simulink model "Current_Fed_DC_DC_Converter_Code_Equivalent_v4"  (R2020a)
settings: Solver=ode3  StartTime=0.0  StopTime=0.4  MaxStep=1e-5  MinStep=1e-7  RelTol=1e-6
InitFcn:
  | %Supply
  | V_supply = 415;
  | f_supply = 50;
  | 
  | %DC_Bus
  | C_filt = 220e-6
  | L_dc = 100e-6;
  | C_out = 560e-3;
  | 
  | %Transformer
  | P_TX = 10e3;
  | V_pri = 36;
  | V_sec = 1;
  | L_leak = 0;
  | R_leak = 0;
  | L_mag = inf;
  | R_mag = inf;
  | 
  | %Control
  | f_sw = 15e3;
  | tss_conv = 0.1;
  | V_ref = 1480;
  | Kp_V = 1;
  | Ki_V = 0.001;
  | I_ref = 2920;
  | Kp_I = 0.025;
  | Ki_I = 0.000001;
  | PS_max = 180;
  | Carr_offset = 1;
  | Carr_scale = 0.5;
  | Duty_scale = 0.01;
  | Duty_fix = 50;
  | Duty_max = 75;
  | Duty_min = 0;
  | f_chop = 1e3;
  | Duty_chop = 40;
  | 
  | %Harmonic_Correction
  | P_inj = 50;
  | f_inj = 50;
  | L_inj = 10e-6;
  | R_inj = 1;
  | Vpri_inj = 1;
  | Vsec_inj = 70;
  | Rleak_inj = 1e-3;
  | Lleak_inj = 12e-6;
  | R_inj = 0.1;
  | Rmag_inj = 1e-3;
  | Lmag_inj = 1e-3;
  | 
  | %Sensor
  | ADC_Res = 4096;
  | I_sense = 1/700;
  | V_sense = 1/50;
  | 
  | %Faults
  | OV_limit = 18.25;
  | UV_limit = 17.5;
  | OC_limit = 515;
  | UC_limit = 22;
  | ... (+3 lines)
libraries: powerlib x109, powerlib_meascontrol x30, simulink x5, slctrlblks x2
(part 2 of 3)

== system Current_Fed_DC_DC_Converter_Code_Equivalent_v4/Module 2/DC DC Converter/DC Bus ==
  DC Bus Parameter : Scope  Commented=on  NumInputPorts=2
  Idc filt : powerlib/Measurements/Current Measurement  PhasorSimulation=off  OutputType=Complex  PSBequivalent=0
  L bus : powerlib/Elements/Series RLC Branch  LConnTagsString=__new0  RConnTagsString=__new0  BranchType=L  Resistance=1  Inductance=L_dc  SetiL0=off  InitialCurrent=0  Capacitance=1e-6  Setx0=off  InitialVoltage=0  Measurements=None
  Vdc : powerlib/Measurements/Voltage Measurement  PhasorSimulation=off  OutputType=Complex  PSBequivalent=0
  +ve IN : PMIOPort  Side=Left
  -ve IN : PMIOPort  Port=2  Side=Left
  +ve OUT : PMIOPort  Port=3  Side=Right
  -ve OUT : PMIOPort  Port=4  Side=Right
  wires:
  Vdc/1 -> DC Bus Parameter/2  "Vdc"
  Idc filt/1 -> DC Bus Parameter/1  "Ifilt"
  connections:
  Idc filt/RConn1 -- +ve OUT/RConn1
  Idc filt/LConn1 -- Vdc/LConn1 -- L bus/RConn1
  Vdc/LConn2 -- -ve IN/RConn1 -- -ve OUT/RConn1
  +ve IN/RConn1 -- L bus/LConn1

== system Current_Fed_DC_DC_Converter_Code_Equivalent_v4/Module 2/DC DC Converter/Filter ==
  C out : powerlib/Elements/Series RLC Branch  LConnTagsString=__new0  RConnTagsString=__new0  BranchType=C  Resistance=10  Inductance=1e-3  SetiL0=off  InitialCurrent=0  Capacitance=C_out  Setx0=off  InitialVoltage=0  Measurements=None
  I C Filter : powerlib/Measurements/Current Measurement  PhasorSimulation=off  OutputType=Complex  PSBequivalent=0
  I out : powerlib/Measurements/Current Measurement  PhasorSimulation=off  OutputType=Complex  PSBequivalent=0
  Output Filter Parameters : Scope  Commented=on  NumInputPorts=2
  +ve IN : PMIOPort  Side=Left
  -ve IN : PMIOPort  Port=2  Side=Left
  +ve OUT : PMIOPort  Port=3  Side=Right
  -ve OUT : PMIOPort  Port=4  Side=Right
  wires:
  I C Filter/1 -> Output Filter Parameters/2
  I out/1 -> Output Filter Parameters/1
  connections:
  +ve OUT/RConn1 -- I out/RConn1
  I C Filter/RConn1 -- C out/LConn1
  I C Filter/LConn1 -- +ve IN/RConn1 -- I out/LConn1
  C out/RConn1 -- -ve OUT/RConn1 -- -ve IN/RConn1

== system Current_Fed_DC_DC_Converter_Code_Equivalent_v4/Module 2/DC DC Converter/HF Transformer ==
  Centre-Tap Transformer 40:1 : powerlib/Elements/Linear Transformer  UNITS=SI  NominalPower=[P_TX f_sw]  winding1=[V_pri R_leak L_leak]  winding2=[V_sec R_leak L_leak]  ThreeWindings=on  winding3=[V_sec R_leak L_leak]  RmLm=[R_mag L_mag]  Measurements=None  DataType=on
  High Frequency Transformer Parameters : Scope  Commented=on  NumInputPorts=5
  Ipri : powerlib/Measurements/Current Measurement  PhasorSimulation=off  OutputType=Complex  PSBequivalent=0
  Isec : powerlib/Measurements/Current Measurement  PhasorSimulation=off  OutputType=Complex  PSBequivalent=0
  Vpri : powerlib/Measurements/Voltage Measurement  PhasorSimulation=off  OutputType=Complex  PSBequivalent=0
  Vsec1 : powerlib/Measurements/Voltage Measurement  PhasorSimulation=off  OutputType=Complex  PSBequivalent=0
  Vsec2 : powerlib/Measurements/Voltage Measurement  PhasorSimulation=off  OutputType=Complex  PSBequivalent=0
  L pri : PMIOPort  Side=Left
  N pri : PMIOPort  Port=2  Side=Left
  L sec : PMIOPort  Port=3  Side=Right
  CT : PMIOPort  Port=4  Side=Right
  N sec : PMIOPort  Port=5  Side=Right
  wires:
  Vpri/1 -> High Frequency Transformer Parameters/5  "V primary"
  Ipri/1 -> High Frequency Transformer Parameters/4  "I primary"
  Vsec2/1 -> High Frequency Transformer Parameters/3  "V secondary 2"
  Vsec1/1 -> High Frequency Transformer Parameters/2  "V secondary 1"
  Isec/1 -> High Frequency Transformer Parameters/1  "I secondary"
  connections:
  Centre-Tap Transformer 40:1/RConn1 -- Vsec1/LConn1 -- Isec/LConn1
  Isec/RConn1 -- L sec/RConn1
  Centre-Tap Transformer 40:1/LConn1 -- Ipri/RConn1
  Centre-Tap Transformer 40:1/RConn4 -- Vsec2/LConn2 -- N sec/RConn1
  Centre-Tap Transformer 40:1/RConn3 -- Centre-Tap Transformer 40:1/RConn2 -- Vsec2/LConn1 -- Vsec1/LConn2 -- CT/RConn1
  Vpri/LConn1 -- L pri/RConn1 -- Ipri/LConn1
  N pri/RConn1 -- Vpri/LConn2 -- Centre-Tap Transformer 40:1/LConn2

== system Current_Fed_DC_DC_Converter_Code_Equivalent_v4/Module 2/DC DC Converter/Inverter ==
  Iref : Inport
  Ifeed : Inport  Port=2
  Vfeed : Inport  Port=3
  Converter : Subsystem
      settings: PortSchema="{\"entries\":[{\"content\":{\"sides\":[{\"content\":{\"connectorIds\":[\"LConn1\",\"LConn2\"]},\"type\":\"ConnectorPlacement.EquallySpacedRectSide\",\"uuid\":\"0645cdc9-e655-49ab-a1d8-1293a5a1d66e\"},{\"content\":{\"connectorIds\":[\"RConn1\",\"RConn2\"],\"side\":\"RIGHT\"},\"type\":\"ConnectorPlacement.EquallySpacedRectSide\",\"uuid\":\"2ef7d2b0-2c84-4192-a188-141ae61cdfda\"},{\"content\":{\"connectorIds\":[\"In1\"],\"side\":\"TOP\"},\"type\":\"ConnectorPlacement.EquallySpacedRectSide\",\"uuid\":\"c5fd5dee-0ba9-4cec-8a2b-47382b263168\"}]},\"type\":\"ConnectorPlacement.EquallySpacedConnector\",\"uuid\":\"4d765392-2146-4c23-badc-b27487fa349e\"}],\"packageUris\":[\"http://schema.mathworks.com/mf0/Connector/19700101\"],\"version\":\"1.0\"}"
  Pulse Generator : Subsystem
  +ve : PMIOPort  Side=Left
  -ve : PMIOPort  Port=2  Side=Left
  Line : PMIOPort  Port=3  Side=Right
  Neutral : PMIOPort  Port=4  Side=Right
  Iref Main : Outport
  wires:
  Iref/1 -> Pulse Generator/1(Iref)
  Pulse Generator/2(Iref Main) -> Iref Main/1
  Ifeed/1 -> Pulse Generator/2(I feed)
  Pulse Generator/1(Pulses) -> Converter/1(Pulses)
  Vfeed/1 -> Pulse Generator/3(V Feed)
  connections:
  Converter/RConn2 -- Neutral/RConn1
  Converter/RConn1 -- Line/RConn1
  Converter/LConn1 -- +ve/RConn1
  Converter/LConn2 -- -ve/RConn1

== system Current_Fed_DC_DC_Converter_Code_Equivalent_v4/Module 2/DC DC Converter/Sensor ==
  Iin : Inport
  Vin : Inport  Port=2
  Current 12bit ADC : Gain  Gain=ADC_Res
  Current Transducer : Gain  Gain=I_sense
  Voltage 12bit ADC : Gain  Gain=ADC_Res
  Voltage Transducer : Gain  Gain=V_sense
  Iout : Outport
  Vout : Outport  Port=2
  wires:
  Vin/1 -> Voltage Transducer/1
  Voltage 12bit ADC/1 -> Vout/1
  Current 12bit ADC/1 -> Iout/1
  Voltage Transducer/1 -> Voltage 12bit ADC/1
  Current Transducer/1 -> Current 12bit ADC/1
  Iin/1 -> Current Transducer/1

== system Current_Fed_DC_DC_Converter_Code_Equivalent_v4/Module 3/3 Phase Rectifier/3 Phase Rectifier ==
  D{1..6} (6 alike) : powerlib/Power Electronics/Diode  Ron=0.001  Lon=0  Vf=0.8  IC=0  UseSnubber=0  Rs=500  Cs=250e-9  Measurements=on
  D1 V&I : Scope  Commented=on
  D2 V&I : Scope  Commented=on
  D3 V&I : Scope  Commented=on
  D4 V&I : Scope  Commented=on
  D5 V&I : Scope  Commented=on
  D6 V&I : Scope  Commented=on
  R Phase : PMIOPort  Side=Left
  Y Phase : PMIOPort  Port=2  Side=Left
  B Phase : PMIOPort  Port=3  Side=Left
  +ve : PMIOPort  Port=4  Side=Right
  -ve : PMIOPort  Port=5  Side=Right
  wires:
  D1/1 -> D1 V&I/1
  D4/1 -> D4 V&I/1
  D3/1 -> D3 V&I/1
  D5/1 -> D5 V&I/1
  D2/1 -> D2 V&I/1
  D6/1 -> D6 V&I/1
  connections:
  B Phase/RConn1 -- D2/RConn1 -- D5/LConn1
  Y Phase/RConn1 -- D4/RConn1 -- D3/LConn1
  -ve/RConn1 -- D2/LConn1 -- D4/LConn1 -- D6/LConn1
  D5/RConn1 -- +ve/RConn1 -- D3/RConn1 -- D1/RConn1
  R Phase/RConn1 -- D6/RConn1 -- D1/LConn1

== system Current_Fed_DC_DC_Converter_Code_Equivalent_v4/Module 3/3 Phase Rectifier/Filter ==
  Cdc 1 : powerlib/Elements/Series RLC Branch  LConnTagsString=__new0  RConnTagsString=__new0  BranchType=C  Resistance=1  Inductance=1e-3  SetiL0=off  InitialCurrent=0  Capacitance=2*C_filt  Setx0=off  InitialVoltage=0  Measurements=None
  Cdc 2 : powerlib/Elements/Series RLC Branch  LConnTagsString=__new0  RConnTagsString=__new0  BranchType=C  Resistance=1  Inductance=1e-3  SetiL0=off  InitialCurrent=0  Capacitance=2*C_filt  Setx0=off  InitialVoltage=0  Measurements=None
  DC Bus Filter Parameters : Scope  NumInputPorts=2
  Iout : powerlib/Measurements/Current Measurement  PhasorSimulation=off  OutputType=Complex  PSBequivalent=0
  Vout : powerlib/Measurements/Voltage Measurement  PhasorSimulation=off  OutputType=Complex  PSBequivalent=0
  +ve IN : PMIOPort  Side=Left
  -ve In : PMIOPort  Port=2  Side=Left
  +ve OUT : PMIOPort  Port=3  Side=Right
  Mid : PMIOPort  Port=4  Side=Right
  -ve OUT : PMIOPort  Port=5  Side=Right
  wires:
  Vout/1 -> DC Bus Filter Parameters/2  "Vout"
  Iout/1 -> DC Bus Filter Parameters/1  "Iout"
  connections:
  Mid/RConn1 -- Cdc 2/LConn1 -- Cdc 1/RConn1
  +ve OUT/RConn1 -- Iout/RConn1
  -ve OUT/RConn1 -- -ve In/RConn1 -- Cdc 2/RConn1 -- Vout/LConn2
  Iout/LConn1 -- +ve IN/RConn1 -- Cdc 1/LConn1 -- Vout/LConn1

== system Current_Fed_DC_DC_Converter_Code_Equivalent_v4/Module 3/DC DC Converter/Centre Tap Rectifier ==
  D1 : powerlib/Power Electronics/Diode  Ron=0.001  Lon=0  Vf=0.8  IC=0  UseSnubber=0  Rs=500  Cs=250e-9  Measurements=on
  D1 V&I : Scope  Commented=on
  D2 : powerlib/Power Electronics/Diode  Ron=0.001  Lon=0  Vf=0.8  IC=0  UseSnubber=0  Rs=500  Cs=250e-9  Measurements=on
  D2 V&I1 : Scope  Commented=on
  Line : PMIOPort  Side=Left
  Centre-tap : PMIOPort  Port=2  Side=Left
  Neutral : PMIOPort  Port=3  Side=Left
  +ve : PMIOPort  Port=4  Side=Right
  -ve : PMIOPort  Port=5  Side=Right
  wires:
  D1/1 -> D1 V&I/1
  D2/1 -> D2 V&I1/1
  connections:
  D1/RConn1 -- +ve/RConn1 -- D2/RConn1
  D1/LConn1 -- Line/RConn1
  D2/LConn1 -- Neutral/RConn1
  -ve/RConn1 -- Centre-tap/RConn1

== system Current_Fed_DC_DC_Converter_Code_Equivalent_v4/Module 3/DC DC Converter/Chopper ==
  Chop Pulse Generator : Subsystem
  Fault Detection : Subsystem
  Io avg : powerlib_meascontrol/Measurements/Mean  Freq=f_supply  Vinit=0  Ts=0
  Iout : powerlib/Measurements/Current Measurement  PhasorSimulation=off  OutputType=Complex  PSBequivalent=0
  Out Parameters : Scope  NumInputPorts=2
  Qchop : powerlib/Power Electronics/IGBT  Ron=0.001  Lon=0  Vf=1  Tf=1e-6  Tt=2e-6  IC=0  Rs=1e5  Cs=inf  Measurements=on
  Qchop V&I : Scope  Commented=on
  Rchop : powerlib/Elements/Series RLC Branch  LConnTagsString=__new0  RConnTagsString=__new0  BranchType=R  Resistance=0.1  Inductance=1e-3  SetiL0=off  InitialCurrent=0  Capacitance=1e-6  Setx0=off  InitialVoltage=0  Measurements=None
  Vo avg : powerlib_meascontrol/Measurements/Mean  Freq=f_supply  Vinit=0  Ts=0
  Vout : powerlib/Measurements/Voltage Measurement  PhasorSimulation=off  OutputType=Complex  PSBequivalent=0
  +ve IN : PMIOPort  Side=Left
  -ve IN : PMIOPort  Port=2  Side=Left
  +ve OUT : PMIOPort  Port=3  Side=Right
  -ve OUT : PMIOPort  Port=4  Side=Right
  Idc avg : Outport
  Vdc avg : Outport  Port=2
  Vdc : Outport  Port=3
  " Idc" : Outport  Port=4
  wires:
  Chop Pulse Generator/1(Chop Pulse) -> Qchop/1
  Vo avg/1 -> Vdc avg/1  "Vo avg"
  Qchop/1 -> Qchop V&I/1
  Iout/1 -> " Idc"/1, Fault Detection/2(I Output), Io avg/1, Out Parameters/1  "Iout"
  Io avg/1 -> Idc avg/1  "Io avg"
  Vout/1 -> Vdc/1, Vo avg/1, Out Parameters/2, Fault Detection/1(V Output)  "Vout"
  Fault Detection/1(OV Fault) -> Chop Pulse Generator/1(Over Voltage Fault)
  connections:
  +ve OUT/RConn1 -- Iout/RConn1 -- Vout/LConn1
  Rchop/LConn1 -- Qchop/RConn1
  Iout/LConn1 -- +ve IN/RConn1 -- Qchop/LConn1
  -ve OUT/RConn1 -- -ve IN/RConn1 -- Rchop/RConn1 -- Vout/LConn2

== system Current_Fed_DC_DC_Converter_Code_Equivalent_v4/Module 3/DC DC Converter/DC Bus ==
  DC Bus Parameter : Scope  Commented=on  NumInputPorts=2
  Idc filt : powerlib/Measurements/Current Measurement  PhasorSimulation=off  OutputType=Complex  PSBequivalent=0
  L bus : powerlib/Elements/Series RLC Branch  LConnTagsString=__new0  RConnTagsString=__new0  BranchType=L  Resistance=1  Inductance=L_dc  SetiL0=off  InitialCurrent=0  Capacitance=1e-6  Setx0=off  InitialVoltage=0  Measurements=None
  Vdc : powerlib/Measurements/Voltage Measurement  PhasorSimulation=off  OutputType=Complex  PSBequivalent=0
  +ve IN : PMIOPort  Side=Left
  -ve IN : PMIOPort  Port=2  Side=Left
  +ve OUT : PMIOPort  Port=3  Side=Right
  -ve OUT : PMIOPort  Port=4  Side=Right
  wires:
  Vdc/1 -> DC Bus Parameter/2  "Vdc"
  Idc filt/1 -> DC Bus Parameter/1  "Ifilt"
  connections:
  Idc filt/RConn1 -- +ve OUT/RConn1
  Idc filt/LConn1 -- Vdc/LConn1 -- L bus/RConn1
  Vdc/LConn2 -- -ve IN/RConn1 -- -ve OUT/RConn1
  +ve IN/RConn1 -- L bus/LConn1

== system Current_Fed_DC_DC_Converter_Code_Equivalent_v4/Module 3/DC DC Converter/Filter ==
  C out : powerlib/Elements/Series RLC Branch  LConnTagsString=__new0  RConnTagsString=__new0  BranchType=C  Resistance=10  Inductance=1e-3  SetiL0=off  InitialCurrent=0  Capacitance=C_out  Setx0=off  InitialVoltage=0  Measurements=None
  I C Filter : powerlib/Measurements/Current Measurement  PhasorSimulation=off  OutputType=Complex  PSBequivalent=0
  I out : powerlib/Measurements/Current Measurement  PhasorSimulation=off  OutputType=Complex  PSBequivalent=0
  Output Filter Parameters : Scope  Commented=on  NumInputPorts=2
  +ve IN : PMIOPort  Side=Left
  -ve IN : PMIOPort  Port=2  Side=Left
  +ve OUT : PMIOPort  Port=3  Side=Right
  -ve OUT : PMIOPort  Port=4  Side=Right
  wires:
  I C Filter/1 -> Output Filter Parameters/2
  I out/1 -> Output Filter Parameters/1
  connections:
  +ve OUT/RConn1 -- I out/RConn1
  I C Filter/RConn1 -- C out/LConn1
  I C Filter/LConn1 -- +ve IN/RConn1 -- I out/LConn1
  C out/RConn1 -- -ve OUT/RConn1 -- -ve IN/RConn1

== system Current_Fed_DC_DC_Converter_Code_Equivalent_v4/Module 3/DC DC Converter/HF Transformer ==
  Centre-Tap Transformer 40:1 : powerlib/Elements/Linear Transformer  UNITS=SI  NominalPower=[P_TX f_sw]  winding1=[V_pri R_leak L_leak]  winding2=[V_sec R_leak L_leak]  ThreeWindings=on  winding3=[V_sec R_leak L_leak]  RmLm=[R_mag L_mag]  Measurements=None  DataType=on
  High Frequency Transformer Parameters : Scope  Commented=on  NumInputPorts=5
  Ipri : powerlib/Measurements/Current Measurement  PhasorSimulation=off  OutputType=Complex  PSBequivalent=0
  Isec : powerlib/Measurements/Current Measurement  PhasorSimulation=off  OutputType=Complex  PSBequivalent=0
  Vpri : powerlib/Measurements/Voltage Measurement  PhasorSimulation=off  OutputType=Complex  PSBequivalent=0
  Vsec1 : powerlib/Measurements/Voltage Measurement  PhasorSimulation=off  OutputType=Complex  PSBequivalent=0
  Vsec2 : powerlib/Measurements/Voltage Measurement  PhasorSimulation=off  OutputType=Complex  PSBequivalent=0
  L pri : PMIOPort  Side=Left
  N pri : PMIOPort  Port=2  Side=Left
  L sec : PMIOPort  Port=3  Side=Right
  CT : PMIOPort  Port=4  Side=Right
  N sec : PMIOPort  Port=5  Side=Right
  wires:
  Vpri/1 -> High Frequency Transformer Parameters/5  "V primary"
  Ipri/1 -> High Frequency Transformer Parameters/4  "I primary"
  Vsec2/1 -> High Frequency Transformer Parameters/3  "V secondary 2"
  Vsec1/1 -> High Frequency Transformer Parameters/2  "V secondary 1"
  Isec/1 -> High Frequency Transformer Parameters/1  "I secondary"
  connections:
  Centre-Tap Transformer 40:1/RConn1 -- Vsec1/LConn1 -- Isec/LConn1
  Isec/RConn1 -- L sec/RConn1
  Centre-Tap Transformer 40:1/LConn1 -- Ipri/RConn1
  Centre-Tap Transformer 40:1/RConn4 -- Vsec2/LConn2 -- N sec/RConn1
  Centre-Tap Transformer 40:1/RConn3 -- Centre-Tap Transformer 40:1/RConn2 -- Vsec2/LConn1 -- Vsec1/LConn2 -- CT/RConn1
  Vpri/LConn1 -- L pri/RConn1 -- Ipri/LConn1
  N pri/RConn1 -- Vpri/LConn2 -- Centre-Tap Transformer 40:1/LConn2

== system Current_Fed_DC_DC_Converter_Code_Equivalent_v4/Module 3/DC DC Converter/Inverter ==
  Iref : Inport
  Ifeed : Inport  Port=2
  Vfeed : Inport  Port=3
  Converter : Subsystem
      settings: PortSchema="{\"entries\":[{\"content\":{\"sides\":[{\"content\":{\"connectorIds\":[\"LConn1\",\"LConn2\"]},\"type\":\"ConnectorPlacement.EquallySpacedRectSide\",\"uuid\":\"0645cdc9-e655-49ab-a1d8-1293a5a1d66e\"},{\"content\":{\"connectorIds\":[\"RConn1\",\"RConn2\"],\"side\":\"RIGHT\"},\"type\":\"ConnectorPlacement.EquallySpacedRectSide\",\"uuid\":\"2ef7d2b0-2c84-4192-a188-141ae61cdfda\"},{\"content\":{\"connectorIds\":[\"In1\"],\"side\":\"TOP\"},\"type\":\"ConnectorPlacement.EquallySpacedRectSide\",\"uuid\":\"c5fd5dee-0ba9-4cec-8a2b-47382b263168\"}]},\"type\":\"ConnectorPlacement.EquallySpacedConnector\",\"uuid\":\"4d765392-2146-4c23-badc-b27487fa349e\"}],\"packageUris\":[\"http://schema.mathworks.com/mf0/Connector/19700101\"],\"version\":\"1.0\"}"
  Pulse Generator : Subsystem
  +ve : PMIOPort  Side=Left
  -ve : PMIOPort  Port=2  Side=Left
  Line : PMIOPort  Port=3  Side=Right
  Neutral : PMIOPort  Port=4  Side=Right
  Iref Main : Outport
  wires:
  Iref/1 -> Pulse Generator/1(Iref)
  Pulse Generator/2(Iref Main) -> Iref Main/1
  Ifeed/1 -> Pulse Generator/2(I feed)
  Pulse Generator/1(Pulses) -> Converter/1(Pulses)
  Vfeed/1 -> Pulse Generator/3(V Feed)
  connections:
  Converter/RConn2 -- Neutral/RConn1
  Converter/RConn1 -- Line/RConn1
  Converter/LConn1 -- +ve/RConn1
  Converter/LConn2 -- -ve/RConn1

== system Current_Fed_DC_DC_Converter_Code_Equivalent_v4/Module 3/DC DC Converter/Sensor ==
  Iin : Inport
  Vin : Inport  Port=2
  Current 12bit ADC : Gain  Gain=ADC_Res
  Current Transducer : Gain  Gain=I_sense
  Voltage 12bit ADC : Gain  Gain=ADC_Res
  Voltage Transducer : Gain  Gain=V_sense
  Iout : Outport
  Vout : Outport  Port=2
  wires:
  Vin/1 -> Voltage Transducer/1
  Voltage 12bit ADC/1 -> Vout/1
  Current 12bit ADC/1 -> Iout/1
  Voltage Transducer/1 -> Voltage 12bit ADC/1
  Current Transducer/1 -> Current 12bit ADC/1
  Iin/1 -> Current Transducer/1

== system Current_Fed_DC_DC_Converter_Code_Equivalent_v4/Module 1/DC DC Converter/Chopper/Chop Pulse Generator ==
  Over Voltage Fault : Inport
  Carrier Bias : Constant  Value=Carr_offset
  Carrier Scaling : Gain  Gain=Carr_scale
  Chopping Carrier : powerlib_meascontrol/Pulse & Signal Generators/Sawtooth Generator  Freq=f_chop  Phase=0  Ts=0
  Chopping Duty Cycle : Constant  Value=Duty_chop
  Chopping Pulse Parameters : Scope  Commented=on  NumInputPorts=4
  Comparator : RelationalOperator  Operator=<=  OutDataTypeStr=boolean  RndMeth=Simplest
  Duty Cycle Scaling : Gain  Gain=Duty_scale
  Fault Condition Check : Logic  IconShape=distinctive  AllPortsSameDT=off  OutDataTypeStr=boolean
  Level Correction : Sum  Inputs=|++
  Chop Pulse : Outport
  wires:
  Chopping Duty Cycle/1 -> Duty Cycle Scaling/1
  Fault Condition Check/1 -> Chop Pulse/1, Chopping Pulse Parameters/4  "Chop Pulse"
  Level Correction/1 -> Carrier Scaling/1
  Duty Cycle Scaling/1 -> Comparator/2
  Carrier Scaling/1 -> Chopping Pulse Parameters/1, Comparator/1  "Chopper Carrier Wave"
  Over Voltage Fault/1 -> Chopping Pulse Parameters/3, Fault Condition Check/2  "Over-voltage Fault"
  Carrier Bias/1 -> Level Correction/2
  Comparator/1 -> Chopping Pulse Parameters/2, Fault Condition Check/1  "Generic Pulse"
  Chopping Carrier/1 -> Level Correction/1

== system Current_Fed_DC_DC_Converter_Code_Equivalent_v4/Module 1/DC DC Converter/Chopper/Fault Detection ==
  V Output : Inport
  I Output : Inport  Port=2
  Constant : Constant  Value=OV_limit
  Constant1 : Constant  Value=UV_limit
  Constant2 : Constant  Value=OC_limit
  Constant3 : Constant  Value=UC_limit
  Faults : Scope  Commented=on  NumInputPorts=4
  GreaterThan : RelationalOperator  OutDataTypeStr=boolean  RndMeth=Simplest
  GreaterThan1 : RelationalOperator  Operator=<=  OutDataTypeStr=boolean  RndMeth=Simplest
  GreaterThan2 : RelationalOperator  OutDataTypeStr=boolean  RndMeth=Simplest
  GreaterThan3 : RelationalOperator  Operator=<=  OutDataTypeStr=boolean  RndMeth=Simplest
  OV Fault : Outport
  wires:
  Constant2/1 -> GreaterThan2/2
  V Output/1 -> GreaterThan1/1, GreaterThan/1
  Constant/1 -> GreaterThan/2
  Constant3/1 -> GreaterThan3/2
  I Output/1 -> GreaterThan2/1, GreaterThan3/1
  GreaterThan3/1 -> Faults/4  "Under Current Fault"
  Constant1/1 -> GreaterThan1/2
  GreaterThan1/1 -> Faults/2  "Under Voltage Fault"
  GreaterThan2/1 -> Faults/3  "Over Current Fault"
  GreaterThan/1 -> OV Fault/1, Faults/1  "Over Voltage Fault"

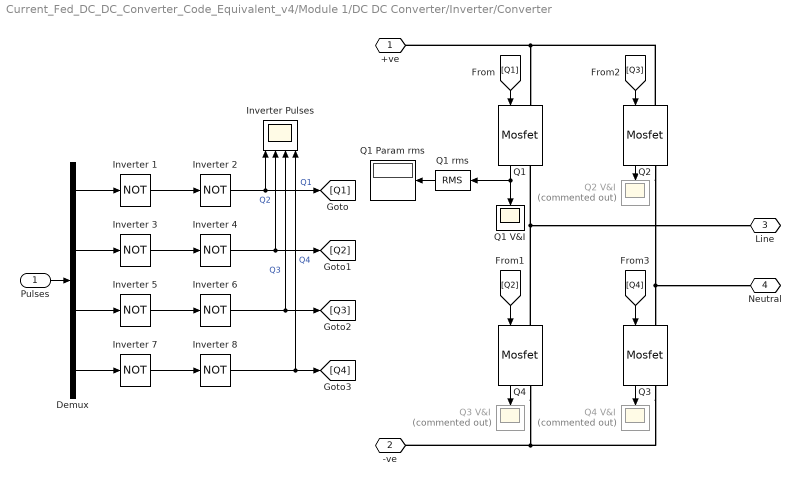
== system Current_Fed_DC_DC_Converter_Code_Equivalent_v4/Module 1/DC DC Converter/Inverter/Converter ==
  Pulses : Inport
  Demux : Demux
  Inverter Pulses : Scope  NumInputPorts=4
  Inverter {1..8} (8 alike) : Logic  Operator=NOT  IconShape=distinctive  AllPortsSameDT=off  OutDataTypeStr=boolean
  Q{1..4} (4 alike) : powerlib/Power Electronics/Mosfet  Ron=0.1  Lon=0  Rd=0.01  Vfd=0  IC=0  Rs=1e5  Cs=inf  Measurements=on
  Q1 V&I : Scope
  Q1 Param rms : Display
  Q1 rms : powerlib_meascontrol/Measurements/RMS  TrueRMS=on  Freq=f_supply  RMSInit=0  Ts=0
  Q2 V&I : Scope  Commented=on
  Q3 V&I : Scope  Commented=on
  Q4 V&I : Scope  Commented=on
  +ve : PMIOPort  Side=Left
  -ve : PMIOPort  Port=2  Side=Left
  Line : PMIOPort  Port=3  Side=Right
  Neutral : PMIOPort  Port=4  Side=Right
  wires:
  Pulses/1 -> Demux/1
  Demux/4 -> Inverter 7/1
  [Q3] -> Q2/1
  [Q1] -> Q1/1
  [Q4] -> Q3/1
  Q4/1 -> Q3 V&I/1
  Q3/1 -> Q4 V&I/1
  [Q2] -> Q4/1
  Demux/2 -> Inverter 3/1
  Q2/1 -> Q2 V&I/1
  Q1/1 -> Q1 rms/1, Q1 V&I/1
  Demux/1 -> Inverter 1/1
  Demux/3 -> Inverter 5/1
  Inverter 1/1 -> Inverter 2/1
  Inverter 8/1 -> [Q4], Inverter Pulses/4  "Q4"
  Inverter 6/1 -> [Q3], Inverter Pulses/3  "Q3"
  Inverter 4/1 -> [Q2], Inverter Pulses/2  "Q2"
  Inverter 2/1 -> [Q1], Inverter Pulses/1  "Q1"
  Inverter 3/1 -> Inverter 4/1
  Inverter 5/1 -> Inverter 6/1
  Inverter 7/1 -> Inverter 8/1
  Q1 rms/1 -> Q1 Param rms/1
  connections:
  Q2/RConn1 -- Neutral/RConn1 -- Q3/LConn1
  Q4/RConn1 -- Q3/RConn1 -- -ve/RConn1
  Q2/LConn1 -- Q1/LConn1 -- +ve/RConn1
  Q4/LConn1 -- Q1/RConn1 -- Line/RConn1

== system Current_Fed_DC_DC_Converter_Code_Equivalent_v4/Module 1/DC DC Converter/Inverter/Pulse Generator ==
  Iref : Inport
  I feed : Inport  Port=2
  V Feed : Inport  Port=3
  Close Loop : Subsystem
  Comparator : Subsystem
  Pulses : Outport
  Iref Main : Outport  Port=2
  wires:
  Comparator/1(Pulses) -> Pulses/1
  Close Loop/1(Phaseshift) -> Comparator/1(Phaseshift)
  V Feed/1 -> Close Loop/3(V Feedback)
  I feed/1 -> Close Loop/2(I Feedback)
  Close Loop/2(Iref Main) -> Iref Main/1
  Iref/1 -> Close Loop/1(Iref)

== system Current_Fed_DC_DC_Converter_Code_Equivalent_v4/Module 2/DC DC Converter/Chopper/Chop Pulse Generator ==
  Over Voltage Fault : Inport
  Carrier Bias : Constant  Value=Carr_offset
  Carrier Scaling : Gain  Gain=Carr_scale
  Chopping Carrier : powerlib_meascontrol/Pulse & Signal Generators/Sawtooth Generator  Freq=f_chop  Phase=0  Ts=0
  Chopping Duty Cycle : Constant  Value=Duty_chop
  Chopping Pulse Parameters : Scope  Commented=on  NumInputPorts=4
  Comparator : RelationalOperator  Operator=<=  OutDataTypeStr=boolean  RndMeth=Simplest
  Duty Cycle Scaling : Gain  Gain=Duty_scale
  Fault Condition Check : Logic  IconShape=distinctive  AllPortsSameDT=off  OutDataTypeStr=boolean
  Level Correction : Sum  Inputs=|++
  Chop Pulse : Outport
  wires:
  Chopping Carrier/1 -> Level Correction/1
  Comparator/1 -> Fault Condition Check/1, Chopping Pulse Parameters/2  "Generic Pulse"
  Carrier Bias/1 -> Level Correction/2
  Over Voltage Fault/1 -> Fault Condition Check/2, Chopping Pulse Parameters/3  "Over-voltage Fault"
  Carrier Scaling/1 -> Comparator/1, Chopping Pulse Parameters/1  "Chopper Carrier Wave"
  Duty Cycle Scaling/1 -> Comparator/2
  Level Correction/1 -> Carrier Scaling/1
  Fault Condition Check/1 -> Chopping Pulse Parameters/4, Chop Pulse/1  "Chop Pulse"
  Chopping Duty Cycle/1 -> Duty Cycle Scaling/1

== system Current_Fed_DC_DC_Converter_Code_Equivalent_v4/Module 2/DC DC Converter/Chopper/Fault Detection ==
  V Output : Inport
  I Output : Inport  Port=2
  Constant : Constant  Value=OV_limit
  Constant1 : Constant  Value=UV_limit
  Constant2 : Constant  Value=OC_limit
  Constant3 : Constant  Value=UC_limit
  Faults : Scope  Commented=on  NumInputPorts=4
  GreaterThan : RelationalOperator  OutDataTypeStr=boolean  RndMeth=Simplest
  GreaterThan1 : RelationalOperator  Operator=<=  OutDataTypeStr=boolean  RndMeth=Simplest
  GreaterThan2 : RelationalOperator  OutDataTypeStr=boolean  RndMeth=Simplest
  GreaterThan3 : RelationalOperator  Operator=<=  OutDataTypeStr=boolean  RndMeth=Simplest
  OV Fault : Outport
  wires:
  GreaterThan/1 -> Faults/1, OV Fault/1  "Over Voltage Fault"
  GreaterThan2/1 -> Faults/3  "Over Current Fault"
  GreaterThan1/1 -> Faults/2  "Under Voltage Fault"
  Constant1/1 -> GreaterThan1/2
  GreaterThan3/1 -> Faults/4  "Under Current Fault"
  I Output/1 -> GreaterThan3/1, GreaterThan2/1
  Constant3/1 -> GreaterThan3/2
  Constant/1 -> GreaterThan/2
  V Output/1 -> GreaterThan/1, GreaterThan1/1
  Constant2/1 -> GreaterThan2/2

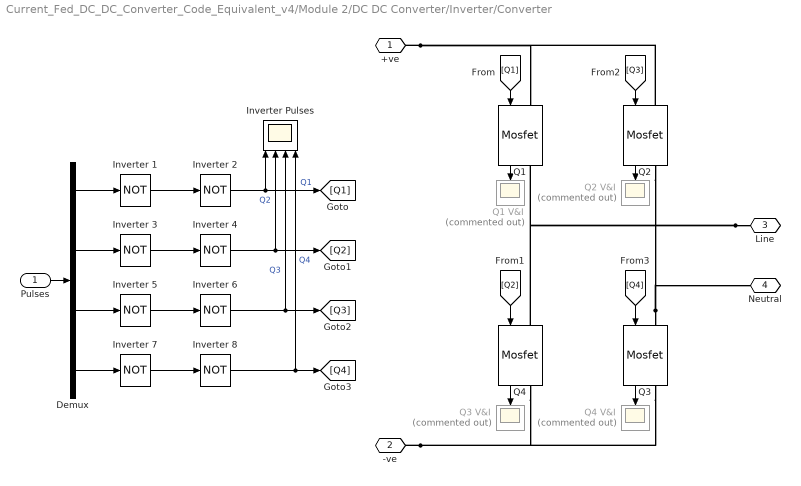
== system Current_Fed_DC_DC_Converter_Code_Equivalent_v4/Module 2/DC DC Converter/Inverter/Converter ==
  Pulses : Inport
  Demux : Demux
  Inverter Pulses : Scope  NumInputPorts=4
  Inverter {1..8} (8 alike) : Logic  Operator=NOT  IconShape=distinctive  AllPortsSameDT=off  OutDataTypeStr=boolean
  Q{1..4} (4 alike) : powerlib/Power Electronics/Mosfet  Ron=0.1  Lon=0  Rd=0.01  Vfd=0  IC=0  Rs=1e5  Cs=inf  Measurements=on
  Q1 V&I : Scope  Commented=on
  Q2 V&I : Scope  Commented=on
  Q3 V&I : Scope  Commented=on
  Q4 V&I : Scope  Commented=on
  +ve : PMIOPort  Side=Left
  -ve : PMIOPort  Port=2  Side=Left
  Line : PMIOPort  Port=3  Side=Right
  Neutral : PMIOPort  Port=4  Side=Right
  wires:
  Inverter 7/1 -> Inverter 8/1
  Inverter 5/1 -> Inverter 6/1
  Inverter 3/1 -> Inverter 4/1
  Inverter 2/1 -> Inverter Pulses/1, [Q1]  "Q1"
  Inverter 4/1 -> Inverter Pulses/2, [Q2]  "Q2"
  Inverter 6/1 -> Inverter Pulses/3, [Q3]  "Q3"
  Inverter 8/1 -> Inverter Pulses/4, [Q4]  "Q4"
  Inverter 1/1 -> Inverter 2/1
  Demux/3 -> Inverter 5/1
  Demux/1 -> Inverter 1/1
  Q1/1 -> Q1 V&I/1
  Q2/1 -> Q2 V&I/1
  Demux/2 -> Inverter 3/1
  [Q2] -> Q4/1
  Q3/1 -> Q4 V&I/1
  Q4/1 -> Q3 V&I/1
  [Q4] -> Q3/1
  [Q1] -> Q1/1
  [Q3] -> Q2/1
  Demux/4 -> Inverter 7/1
  Pulses/1 -> Demux/1
  connections:
  Line/RConn1 -- Q1/RConn1 -- Q4/LConn1
  +ve/RConn1 -- Q1/LConn1 -- Q2/LConn1
  -ve/RConn1 -- Q3/RConn1 -- Q4/RConn1
  Q3/LConn1 -- Neutral/RConn1 -- Q2/RConn1

== system Current_Fed_DC_DC_Converter_Code_Equivalent_v4/Module 2/DC DC Converter/Inverter/Pulse Generator ==
  Iref : Inport
  I feed : Inport  Port=2
  V Feed : Inport  Port=3
  Close Loop : Subsystem
  Comparator : Subsystem
  Pulses : Outport
  Iref Main : Outport  Port=2
  wires:
  Iref/1 -> Close Loop/1(Iref)
  Close Loop/2(Iref Main) -> Iref Main/1
  I feed/1 -> Close Loop/2(I Feedback)
  V Feed/1 -> Close Loop/3(V Feedback)
  Close Loop/1(Phaseshift) -> Comparator/1(Phaseshift)
  Comparator/1(Pulses) -> Pulses/1

== system Current_Fed_DC_DC_Converter_Code_Equivalent_v4/Module 3/DC DC Converter/Chopper/Chop Pulse Generator ==
  Over Voltage Fault : Inport
  Carrier Bias : Constant  Value=Carr_offset
  Carrier Scaling : Gain  Gain=Carr_scale
  Chopping Carrier : powerlib_meascontrol/Pulse & Signal Generators/Sawtooth Generator  Freq=f_chop  Phase=0  Ts=0
  Chopping Duty Cycle : Constant  Value=Duty_chop
  Chopping Pulse Parameters : Scope  Commented=on  NumInputPorts=4
  Comparator : RelationalOperator  Operator=<=  OutDataTypeStr=boolean  RndMeth=Simplest
  Duty Cycle Scaling : Gain  Gain=Duty_scale
  Fault Condition Check : Logic  IconShape=distinctive  AllPortsSameDT=off  OutDataTypeStr=boolean
  Level Correction : Sum  Inputs=|++
  Chop Pulse : Outport
  wires:
  Chopping Carrier/1 -> Level Correction/1
  Comparator/1 -> Fault Condition Check/1, Chopping Pulse Parameters/2  "Generic Pulse"
  Carrier Bias/1 -> Level Correction/2
  Over Voltage Fault/1 -> Fault Condition Check/2, Chopping Pulse Parameters/3  "Over-voltage Fault"
  Carrier Scaling/1 -> Comparator/1, Chopping Pulse Parameters/1  "Chopper Carrier Wave"
  Duty Cycle Scaling/1 -> Comparator/2
  Level Correction/1 -> Carrier Scaling/1
  Fault Condition Check/1 -> Chopping Pulse Parameters/4, Chop Pulse/1  "Chop Pulse"
  Chopping Duty Cycle/1 -> Duty Cycle Scaling/1

== system Current_Fed_DC_DC_Converter_Code_Equivalent_v4/Module 3/DC DC Converter/Chopper/Fault Detection ==
  V Output : Inport
  I Output : Inport  Port=2
  Constant : Constant  Value=OV_limit
  Constant1 : Constant  Value=UV_limit
  Constant2 : Constant  Value=OC_limit
  Constant3 : Constant  Value=UC_limit
  Faults : Scope  Commented=on  NumInputPorts=4
  GreaterThan : RelationalOperator  OutDataTypeStr=boolean  RndMeth=Simplest
  GreaterThan1 : RelationalOperator  Operator=<=  OutDataTypeStr=boolean  RndMeth=Simplest
  GreaterThan2 : RelationalOperator  OutDataTypeStr=boolean  RndMeth=Simplest
  GreaterThan3 : RelationalOperator  Operator=<=  OutDataTypeStr=boolean  RndMeth=Simplest
  OV Fault : Outport
  wires:
  GreaterThan/1 -> Faults/1, OV Fault/1  "Over Voltage Fault"
  GreaterThan2/1 -> Faults/3  "Over Current Fault"
  GreaterThan1/1 -> Faults/2  "Under Voltage Fault"
  Constant1/1 -> GreaterThan1/2
  GreaterThan3/1 -> Faults/4  "Under Current Fault"
  I Output/1 -> GreaterThan3/1, GreaterThan2/1
  Constant3/1 -> GreaterThan3/2
  Constant/1 -> GreaterThan/2
  V Output/1 -> GreaterThan/1, GreaterThan1/1
  Constant2/1 -> GreaterThan2/2

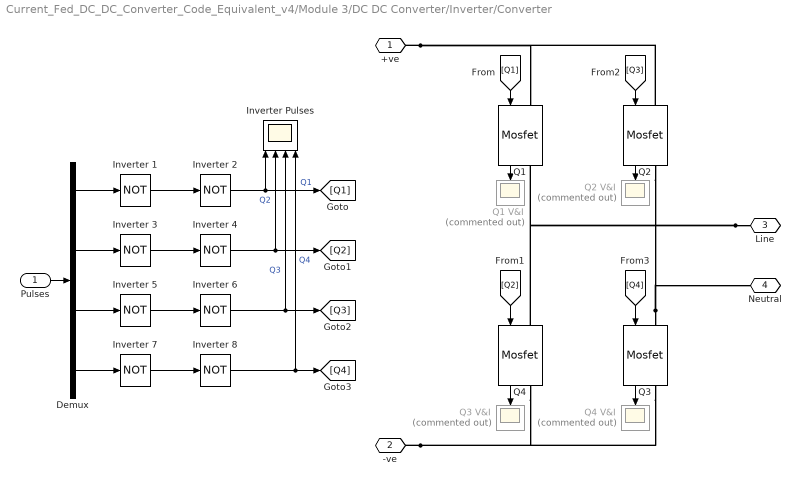
== system Current_Fed_DC_DC_Converter_Code_Equivalent_v4/Module 3/DC DC Converter/Inverter/Converter ==
  Pulses : Inport
  Demux : Demux
  Inverter Pulses : Scope  NumInputPorts=4
  Inverter {1..8} (8 alike) : Logic  Operator=NOT  IconShape=distinctive  AllPortsSameDT=off  OutDataTypeStr=boolean
  Q{1..4} (4 alike) : powerlib/Power Electronics/Mosfet  Ron=0.1  Lon=0  Rd=0.01  Vfd=0  IC=0  Rs=1e5  Cs=inf  Measurements=on
  Q1 V&I : Scope  Commented=on
  Q2 V&I : Scope  Commented=on
  Q3 V&I : Scope  Commented=on
  Q4 V&I : Scope  Commented=on
  +ve : PMIOPort  Side=Left
  -ve : PMIOPort  Port=2  Side=Left
  Line : PMIOPort  Port=3  Side=Right
  Neutral : PMIOPort  Port=4  Side=Right
  wires:
  Inverter 7/1 -> Inverter 8/1
  Inverter 5/1 -> Inverter 6/1
  Inverter 3/1 -> Inverter 4/1
  Inverter 2/1 -> Inverter Pulses/1, [Q1]  "Q1"
  Inverter 4/1 -> Inverter Pulses/2, [Q2]  "Q2"
  Inverter 6/1 -> Inverter Pulses/3, [Q3]  "Q3"
  Inverter 8/1 -> Inverter Pulses/4, [Q4]  "Q4"
  Inverter 1/1 -> Inverter 2/1
  Demux/3 -> Inverter 5/1
  Demux/1 -> Inverter 1/1
  Q1/1 -> Q1 V&I/1
  Q2/1 -> Q2 V&I/1
  Demux/2 -> Inverter 3/1
  [Q2] -> Q4/1
  Q3/1 -> Q4 V&I/1
  Q4/1 -> Q3 V&I/1
  [Q4] -> Q3/1
  [Q1] -> Q1/1
  [Q3] -> Q2/1
  Demux/4 -> Inverter 7/1
  Pulses/1 -> Demux/1
  connections:
  Line/RConn1 -- Q1/RConn1 -- Q4/LConn1
  +ve/RConn1 -- Q1/LConn1 -- Q2/LConn1
  -ve/RConn1 -- Q3/RConn1 -- Q4/RConn1
  Q3/LConn1 -- Neutral/RConn1 -- Q2/RConn1

== system Current_Fed_DC_DC_Converter_Code_Equivalent_v4/Module 3/DC DC Converter/Inverter/Pulse Generator ==
  Iref : Inport
  I feed : Inport  Port=2
  V Feed : Inport  Port=3
  Close Loop : Subsystem
  Comparator : Subsystem
  Pulses : Outport
  Iref Main : Outport  Port=2
  wires:
  Iref/1 -> Close Loop/1(Iref)
  Close Loop/2(Iref Main) -> Iref Main/1
  I feed/1 -> Close Loop/2(I Feedback)
  V Feed/1 -> Close Loop/3(V Feedback)
  Close Loop/1(Phaseshift) -> Comparator/1(Phaseshift)
  Comparator/1(Pulses) -> Pulses/1

== system Current_Fed_DC_DC_Converter_Code_Equivalent_v4/Module 1/DC DC Converter/Inverter/Pulse Generator/Close Loop ==
  Iref : Inport
  I Feedback : Inport  Port=2
  V Feedback : Inport  Port=3
  Current Loop : Subsystem
  Duty Cycle : Display
  I Reference : Display
  Iout avg : Display
  Master/Slave Select : ManualSwitch
  Voltage Loop : Subsystem
  Vout avg : Display
  Phaseshift : Outport
  Iref Main : Outport  Port=2
  wires:
  V Feedback/1 -> Vout avg/1, Voltage Loop/1(V Feedback)  "Vfbk"
  I Feedback/1 -> Iout avg/1, Current Loop/2(I Feedback)  "Ifbk"
  Current Loop/1(PI Out) -> Duty Cycle/1, Phaseshift/1
  Master/Slave Select/1 -> Iref Main/1, I Reference/1, Current Loop/1(I Reference)  "Iref"
  Iref/1 -> Master/Slave Select/2
  Voltage Loop/1(PI Out) -> Master/Slave Select/1  "V PI Out"

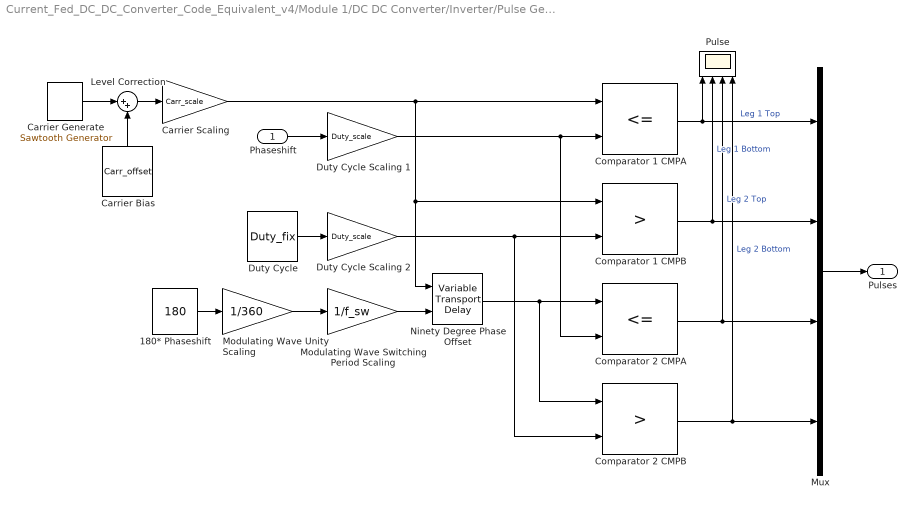
== system Current_Fed_DC_DC_Converter_Code_Equivalent_v4/Module 1/DC DC Converter/Inverter/Pulse Generator/Comparator ==
  Phaseshift : Inport
  180* Phaseshift : Constant  Value=180
  Carrier Bias : Constant  Value=Carr_offset
  Carrier Generate : powerlib_meascontrol/Pulse & Signal Generators/Sawtooth Generator  Freq=f_sw  Phase=0  Ts=0
  Carrier Scaling : Gain  Gain=Carr_scale
  Comparator 1 CMPA : RelationalOperator  Operator=<=  OutDataTypeStr=boolean  RndMeth=Simplest
  Comparator 1 CMPB : RelationalOperator  Operator=>  OutDataTypeStr=boolean  RndMeth=Simplest
  Comparator 2 CMPA : RelationalOperator  Operator=<=  OutDataTypeStr=boolean  RndMeth=Simplest
  Comparator 2 CMPB : RelationalOperator  Operator=>  OutDataTypeStr=boolean  RndMeth=Simplest
  Duty Cycle : Constant  Value=Duty_fix
  Duty Cycle Scaling 1 : Gain  Gain=Duty_scale
  Duty Cycle Scaling 2 : Gain  Gain=Duty_scale
  Level Correction : Sum  Inputs=|++
  Modulating Wave Switching Period Scaling : Gain  Gain=1/f_sw
  Modulating Wave Unity Scaling : Gain  Gain=1/360
  Mux : Mux
  Ninety Degree Phase Offset : VariableTransportDelay  MaximumDelay=(PS_max/360)*(1/f_sw)  MaximumPoints=131072
  Pulse : Scope  NumInputPorts=4
  Pulses : Outport
  wires:
  Duty Cycle Scaling 1/1 -> Comparator 2 CMPA/2, Comparator 1 CMPA/2
  Phaseshift/1 -> Duty Cycle Scaling 1/1
  Modulating Wave Switching Period Scaling/1 -> Ninety Degree Phase Offset/2
  Modulating Wave Unity Scaling/1 -> Modulating Wave Switching Period Scaling/1
  180* Phaseshift/1 -> Modulating Wave Unity Scaling/1
  Carrier Generate/1 -> Level Correction/1
  Carrier Bias/1 -> Level Correction/2
  Duty Cycle/1 -> Duty Cycle Scaling 2/1
  Level Correction/1 -> Carrier Scaling/1
  Carrier Scaling/1 -> Ninety Degree Phase Offset/1, Comparator 1 CMPB/1, Comparator 1 CMPA/1
  Comparator 1 CMPA/1 -> Mux/1, Pulse/1  "Leg 1 Top"
  Mux/1 -> Pulses/1
  Duty Cycle Scaling 2/1 -> Comparator 2 CMPB/2, Comparator 1 CMPB/2
  Ninety Degree Phase Offset/1 -> Comparator 2 CMPA/1, Comparator 2 CMPB/1
  Comparator 1 CMPB/1 -> Mux/2, Pulse/2  "Leg 1 Bottom"
  Comparator 2 CMPA/1 -> Mux/3, Pulse/3  "Leg 2 Top"
  Comparator 2 CMPB/1 -> Mux/4, Pulse/4  "Leg 2 Bottom"

== system Current_Fed_DC_DC_Converter_Code_Equivalent_v4/Module 2/DC DC Converter/Inverter/Pulse Generator/Close Loop ==
  Iref : Inport
  I Feedback : Inport  Port=2
  V Feedback : Inport  Port=3
  Current Loop : Subsystem
  Duty Cycle : Display
  I Reference : Display
  Iout avg : Display
  Master/Slave Select : ManualSwitch  CurrentSetting=0
  Voltage Loop : Subsystem
  Vout avg : Display
  Phaseshift : Outport
  Iref Main : Outport  Port=2
  wires:
  Voltage Loop/1(PI Out) -> Master/Slave Select/1  "V PI Out"
  Iref/1 -> Master/Slave Select/2
  Master/Slave Select/1 -> Current Loop/1(I Reference), I Reference/1, Iref Main/1  "Iref"
  Current Loop/1(PI Out) -> Phaseshift/1, Duty Cycle/1
  I Feedback/1 -> Current Loop/2(I Feedback), Iout avg/1  "Ifbk"
  V Feedback/1 -> Voltage Loop/1(V Feedback), Vout avg/1  "Vfbk"

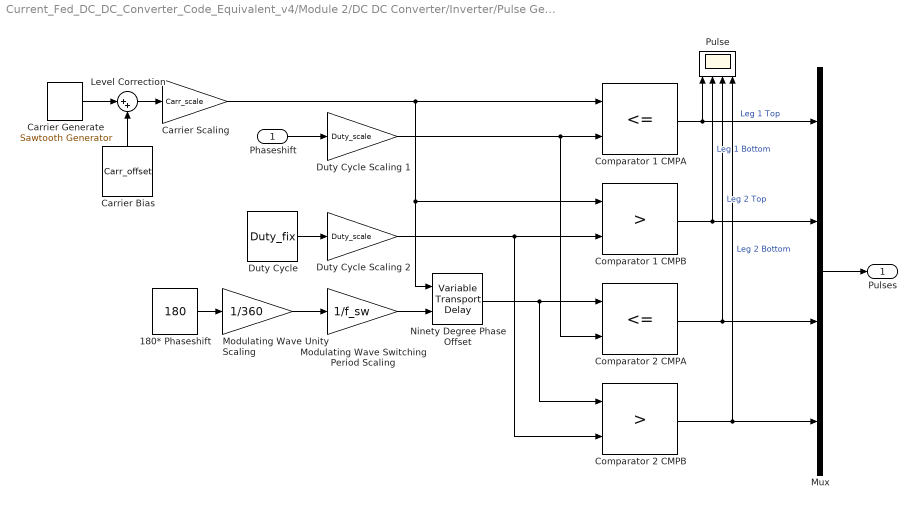
== system Current_Fed_DC_DC_Converter_Code_Equivalent_v4/Module 2/DC DC Converter/Inverter/Pulse Generator/Comparator ==
  Phaseshift : Inport
  180* Phaseshift : Constant  Value=180
  Carrier Bias : Constant  Value=Carr_offset
  Carrier Generate : powerlib_meascontrol/Pulse & Signal Generators/Sawtooth Generator  Freq=f_sw  Phase=0  Ts=0
  Carrier Scaling : Gain  Gain=Carr_scale
  Comparator 1 CMPA : RelationalOperator  Operator=<=  OutDataTypeStr=boolean  RndMeth=Simplest
  Comparator 1 CMPB : RelationalOperator  Operator=>  OutDataTypeStr=boolean  RndMeth=Simplest
  Comparator 2 CMPA : RelationalOperator  Operator=<=  OutDataTypeStr=boolean  RndMeth=Simplest
  Comparator 2 CMPB : RelationalOperator  Operator=>  OutDataTypeStr=boolean  RndMeth=Simplest
  Duty Cycle : Constant  Value=Duty_fix
  Duty Cycle Scaling 1 : Gain  Gain=Duty_scale
  Duty Cycle Scaling 2 : Gain  Gain=Duty_scale
  Level Correction : Sum  Inputs=|++
  Modulating Wave Switching Period Scaling : Gain  Gain=1/f_sw
  Modulating Wave Unity Scaling : Gain  Gain=1/360
  Mux : Mux
  Ninety Degree Phase Offset : VariableTransportDelay  MaximumDelay=(PS_max/360)*(1/f_sw)  MaximumPoints=131072
  Pulse : Scope  NumInputPorts=4
  Pulses : Outport
  wires:
  Comparator 2 CMPB/1 -> Pulse/4, Mux/4  "Leg 2 Bottom"
  Comparator 2 CMPA/1 -> Pulse/3, Mux/3  "Leg 2 Top"
  Comparator 1 CMPB/1 -> Pulse/2, Mux/2  "Leg 1 Bottom"
  Ninety Degree Phase Offset/1 -> Comparator 2 CMPB/1, Comparator 2 CMPA/1
  Duty Cycle Scaling 2/1 -> Comparator 1 CMPB/2, Comparator 2 CMPB/2
  Mux/1 -> Pulses/1
  Comparator 1 CMPA/1 -> Pulse/1, Mux/1  "Leg 1 Top"
  Carrier Scaling/1 -> Comparator 1 CMPA/1, Comparator 1 CMPB/1, Ninety Degree Phase Offset/1
  Level Correction/1 -> Carrier Scaling/1
  Duty Cycle/1 -> Duty Cycle Scaling 2/1
  Carrier Bias/1 -> Level Correction/2
  Carrier Generate/1 -> Level Correction/1
  180* Phaseshift/1 -> Modulating Wave Unity Scaling/1
  Modulating Wave Unity Scaling/1 -> Modulating Wave Switching Period Scaling/1
  Modulating Wave Switching Period Scaling/1 -> Ninety Degree Phase Offset/2
  Phaseshift/1 -> Duty Cycle Scaling 1/1
  Duty Cycle Scaling 1/1 -> Comparator 1 CMPA/2, Comparator 2 CMPA/2

== system Current_Fed_DC_DC_Converter_Code_Equivalent_v4/Module 3/DC DC Converter/Inverter/Pulse Generator/Close Loop ==
  Iref : Inport
  I Feedback : Inport  Port=2
  V Feedback : Inport  Port=3
  Current Loop : Subsystem
  Duty Cycle : Display
  I Reference : Display
  Iout avg : Display
  Master/Slave Select : ManualSwitch  CurrentSetting=0
  Voltage Loop : Subsystem
  Vout avg : Display
  Phaseshift : Outport
  Iref Main : Outport  Port=2
  wires:
  Voltage Loop/1(PI Out) -> Master/Slave Select/1  "V PI Out"
  Iref/1 -> Master/Slave Select/2
  Master/Slave Select/1 -> Current Loop/1(I Reference), I Reference/1, Iref Main/1  "Iref"
  Current Loop/1(PI Out) -> Phaseshift/1, Duty Cycle/1
  I Feedback/1 -> Current Loop/2(I Feedback), Iout avg/1  "Ifbk"
  V Feedback/1 -> Voltage Loop/1(V Feedback), Vout avg/1  "Vfbk"

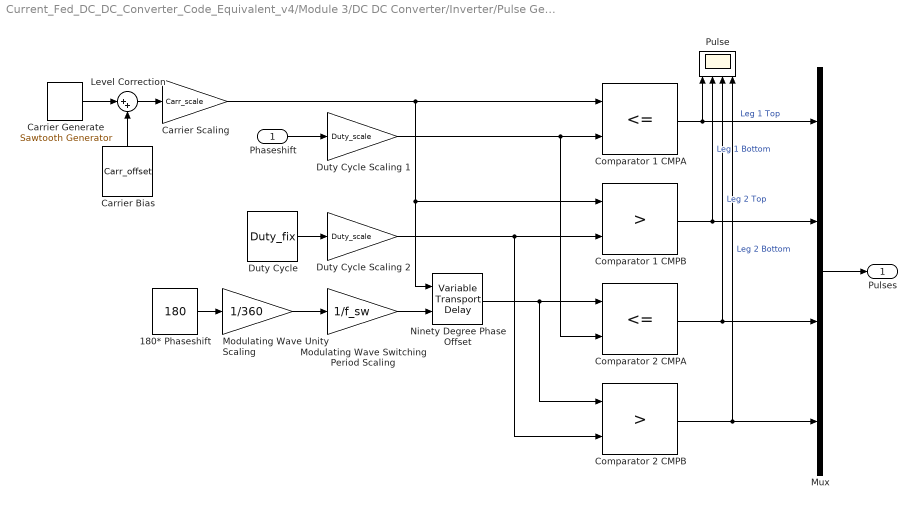
== system Current_Fed_DC_DC_Converter_Code_Equivalent_v4/Module 3/DC DC Converter/Inverter/Pulse Generator/Comparator ==
  Phaseshift : Inport
  180* Phaseshift : Constant  Value=180
  Carrier Bias : Constant  Value=Carr_offset
  Carrier Generate : powerlib_meascontrol/Pulse & Signal Generators/Sawtooth Generator  Freq=f_sw  Phase=0  Ts=0
  Carrier Scaling : Gain  Gain=Carr_scale
  Comparator 1 CMPA : RelationalOperator  Operator=<=  OutDataTypeStr=boolean  RndMeth=Simplest
  Comparator 1 CMPB : RelationalOperator  Operator=>  OutDataTypeStr=boolean  RndMeth=Simplest
  Comparator 2 CMPA : RelationalOperator  Operator=<=  OutDataTypeStr=boolean  RndMeth=Simplest
  Comparator 2 CMPB : RelationalOperator  Operator=>  OutDataTypeStr=boolean  RndMeth=Simplest
  Duty Cycle : Constant  Value=Duty_fix
  Duty Cycle Scaling 1 : Gain  Gain=Duty_scale
  Duty Cycle Scaling 2 : Gain  Gain=Duty_scale
  Level Correction : Sum  Inputs=|++
  Modulating Wave Switching Period Scaling : Gain  Gain=1/f_sw
  Modulating Wave Unity Scaling : Gain  Gain=1/360
  Mux : Mux
  Ninety Degree Phase Offset : VariableTransportDelay  MaximumDelay=(PS_max/360)*(1/f_sw)  MaximumPoints=131072
  Pulse : Scope  NumInputPorts=4
  Pulses : Outport
  wires:
  Comparator 2 CMPB/1 -> Pulse/4, Mux/4  "Leg 2 Bottom"
  Comparator 2 CMPA/1 -> Pulse/3, Mux/3  "Leg 2 Top"
  Comparator 1 CMPB/1 -> Pulse/2, Mux/2  "Leg 1 Bottom"
  Ninety Degree Phase Offset/1 -> Comparator 2 CMPB/1, Comparator 2 CMPA/1
  Duty Cycle Scaling 2/1 -> Comparator 1 CMPB/2, Comparator 2 CMPB/2
  Mux/1 -> Pulses/1
  Comparator 1 CMPA/1 -> Pulse/1, Mux/1  "Leg 1 Top"
  Carrier Scaling/1 -> Comparator 1 CMPA/1, Comparator 1 CMPB/1, Ninety Degree Phase Offset/1
  Level Correction/1 -> Carrier Scaling/1
  Duty Cycle/1 -> Duty Cycle Scaling 2/1
  Carrier Bias/1 -> Level Correction/2
  Carrier Generate/1 -> Level Correction/1
  180* Phaseshift/1 -> Modulating Wave Unity Scaling/1
  Modulating Wave Unity Scaling/1 -> Modulating Wave Switching Period Scaling/1
  Modulating Wave Switching Period Scaling/1 -> Ninety Degree Phase Offset/2
  Phaseshift/1 -> Duty Cycle Scaling 1/1
  Duty Cycle Scaling 1/1 -> Comparator 1 CMPA/2, Comparator 2 CMPA/2

== system Current_Fed_DC_DC_Converter_Code_Equivalent_v4/Module 1/DC DC Converter/Inverter/Pulse Generator/Close Loop/Current Loop ==
  I Reference : Inport
  I Feedback : Inport  Port=2
  Current PI Parmaters : Scope  NumInputPorts=8
  Error : Sum  Inputs=|+-
  Integrate : Sum  Inputs=|++
  Ki : Gain  Gain=Ki_I
  Kp : Gain  Gain=Kp_I
  PI : Sum  Inputs=|++
  PI Clamp : Saturate  UpperLimit=Duty_max  LowerLimit=Duty_min
  Previous Value : UnitDelay  SampleTime=-1  HasFrameUpgradeWarning=on
  Reference Clamp : Saturate  UpperLimit=I_ref  LowerLimit=0
  PI Out : Outport
  wires:
  Previous Value/1 -> Current PI Parmaters/4, Integrate/2  "I Error Previous"
  Kp/1 -> PI/1, Current PI Parmaters/5  "Proportional Out"
  Ki/1 -> PI/2, Current PI Parmaters/6  "Integral Out"
  Integrate/1 -> Ki/1, Previous Value/1
  Error/1 -> Kp/1, Current PI Parmaters/3, Integrate/1  "I Error"
  I Reference/1 -> Reference Clamp/1  "I Reference"
  I Feedback/1 -> Error/2, Current PI Parmaters/2  "I Feedback"
  PI Clamp/1 -> PI Out/1, Current PI Parmaters/8  "Duty Cycle Clamped"
  PI/1 -> PI Clamp/1, Current PI Parmaters/7  "Duty Cycle Shift"
  Reference Clamp/1 -> Current PI Parmaters/1, Error/1  "PI Saturated"

== system Current_Fed_DC_DC_Converter_Code_Equivalent_v4/Module 1/DC DC Converter/Inverter/Pulse Generator/Close Loop/Voltage Loop ==
  V Feedback : Inport
  Error : Sum  Inputs=|+-
  Integration : Sum  Inputs=|++
  Ki : Gain  Gain=Ki_V
  Kp : Gain  Gain=Kp_V
  PI Clamp : Saturate  UpperLimit=I_ref  LowerLimit=0
  PI Output : Sum  Inputs=|++
  Previous Value : UnitDelay  SampleTime=-1  HasFrameUpgradeWarning=on
  SoftStart Ramp : simulink/Sources/Ramp  slope=V_ref/tss_conv  start=0  InitialOutput=0
  V Reference : Saturate  UpperLimit=V_ref  LowerLimit=0
  Voltage PI Parmaters : Scope  NumInputPorts=9
  PI Out : Outport
  wires:
  Integration/1 -> Previous Value/1, Ki/1
  Previous Value/1 -> Voltage PI Parmaters/5, Integration/2  "V Error Previous"
  Kp/1 -> PI Output/1, Voltage PI Parmaters/6  "Proportional Out"
  V Feedback/1 -> Error/2, Voltage PI Parmaters/3  "V Feedback"
  PI Output/1 -> PI Clamp/1, Voltage PI Parmaters/8  "PI Out"
  Error/1 -> Kp/1, Voltage PI Parmaters/4, Integration/1  "V Error"
  Ki/1 -> PI Output/2, Voltage PI Parmaters/7  "Integral Out"
  V Reference/1 -> Error/1, Voltage PI Parmaters/2  "V Reference"
  SoftStart Ramp/1 -> V Reference/1, Voltage PI Parmaters/1  "V Reference Ramp"
  PI Clamp/1 -> PI Out/1, Voltage PI Parmaters/9  "PI Saturated"

== system Current_Fed_DC_DC_Converter_Code_Equivalent_v4/Module 2/DC DC Converter/Inverter/Pulse Generator/Close Loop/Current Loop ==
  I Reference : Inport
  I Feedback : Inport  Port=2
  Current PI Parmaters : Scope  NumInputPorts=8
  Error : Sum  Inputs=|+-
  Integrate : Sum  Inputs=|++
  Ki : Gain  Gain=Ki_I
  Kp : Gain  Gain=Kp_I
  PI : Sum  Inputs=|++
  PI Clamp : Saturate  UpperLimit=Duty_max  LowerLimit=Duty_min
  Previous Value : UnitDelay  SampleTime=-1  HasFrameUpgradeWarning=on
  Reference Clamp : Saturate  UpperLimit=I_ref  LowerLimit=0
  PI Out : Outport
  wires:
  Reference Clamp/1 -> Error/1, Current PI Parmaters/1  "PI Saturated"
  PI/1 -> Current PI Parmaters/7, PI Clamp/1  "Duty Cycle Shift"
  PI Clamp/1 -> Current PI Parmaters/8, PI Out/1  "Duty Cycle Clamped"
  I Feedback/1 -> Current PI Parmaters/2, Error/2  "I Feedback"
  I Reference/1 -> Reference Clamp/1  "I Reference"
  Error/1 -> Integrate/1, Current PI Parmaters/3, Kp/1  "I Error"
  Integrate/1 -> Previous Value/1, Ki/1
  Ki/1 -> Current PI Parmaters/6, PI/2  "Integral Out"
  Kp/1 -> Current PI Parmaters/5, PI/1  "Proportional Out"
  Previous Value/1 -> Integrate/2, Current PI Parmaters/4  "I Error Previous"
